simulink model "ac_monitor_A_test"  (R2024b)
settings: Solver=VariableStepAuto  StartTime=0.0  StopTime=80  RelTol=1e-3
PreLoadFcn:
  | load_system('../simulink_reference_models/test_sequence_lib');
InitFcn:
  | close all
  | clear all
  | 
  | T_CNTL = 1/5e3;
  | 
  | VLL_NOM = 35e3;
  | F_NOM = 60;
libraries: test_sequence_lib x4
settings Model: SimulationMode=rapid-accelerator  Creator=HussamAlatrash  LastModifiedBy=ritvik_heron

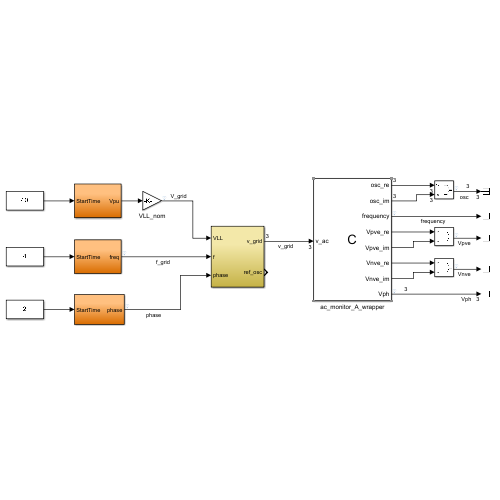
[thumbnail: Simulink's stored preview of the top-level diagram]
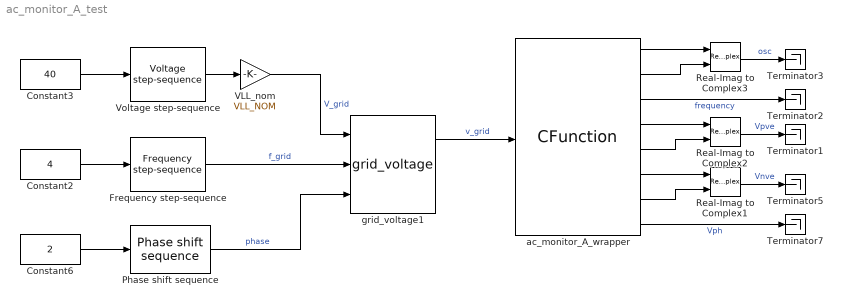
== system ac_monitor_A_test ==
  Constant2 : Constant  Value=4
  Constant3 : Constant  Value=40
  Constant6 : Constant  Value=2
  Frequency step-sequence : test_sequence_lib/Frequency step-sequence  SystemSampleTime=-1  VariantActivationTime=update diagram  AllowFlexibleInterface=on  Latency=0  AutoFrameSizeCalculation=off
  Phase shift sequence : test_sequence_lib/Phase shift sequence  SystemSampleTime=-1  VariantActivationTime=update diagram  AllowFlexibleInterface=on  Latency=0  AutoFrameSizeCalculation=off
  Real-Imag to Complex1 : RealImagToComplex
  Real-Imag to Complex2 : RealImagToComplex
  Real-Imag to Complex3 : RealImagToComplex
  Terminator{1..3,5,7} (5 alike) : Terminator
  VLL_nom : Gain  Gain=VLL_NOM
  Voltage step-sequence : test_sequence_lib/Voltage step-sequence  SystemSampleTime=-1  VariantActivationTime=update diagram  AllowFlexibleInterface=on  Latency=0  AutoFrameSizeCalculation=off
  ac_monitor_A_wrapper : CFunction  OutputCode=|  StartCode=|  CodegenOutputCode=|  CodegenStartCode=|  SampleTime=200e-6  SimCustomHeaderFile=../c_language_library/companion_algorithms/ac_monitor_A/acMonitor_A_autogen.h  SimCustomSourceFile=../c_language_library/companion_algorithms/ac_monitor_A/ac_monitor_A.c ../c_language_library/helper_lib/cmplx.c  CustomHeaderFile=../c_language_library/companion_algorithms/ac_monitor_A/acMonitor_A_autogen.h  CustomSourceFile=../c_language_library/companion_algorithms/ac_monitor_A/ac_monitor_A.c ../c_language_library/helper_lib/cmplx.c
      OutputCode=|
      | acMonitor_IN.v_ac[0] = v_ac[0];
      | acMonitor_IN.v_ac[1] = v_ac[1];
      | acMonitor_IN.v_ac[2] = v_ac[2];
      | 
      | 
      | acMonitor_5kHz(200e-6f);
      | 
      | osc_re[0] = acMonitor_OUT.pll_osc[0].real;
      | osc_im[0] = acMonitor_OUT.pll_osc[0].imag;
      | osc_re[1] = acMonitor_OUT.pll_osc[1].real;
      | osc_im[1] = acMonitor_OUT.pll_osc[1].imag;
      | osc_re[2] = acMonitor_OUT.pll_osc[2].real;
      | osc_im[2] = acMonitor_OUT.pll_osc[2].imag;
      | 
      | frequency = acMonitor_OUT.frequency;
      | Vpve_re = acMonitor_OUT.Vpve.real;
      | Vpve_im = acMonitor_OUT.Vpve.imag;
      | Vnve_re = acMonitor_OUT.Vnve.real;
      | Vnve_im = acMonitor_OUT.Vnve.imag;
      | 
      | Vph[0] = acMonitor_OUT.Vph[0];
      | Vph[1] = acMonitor_OUT.Vph[1];
      | Vph[2] = acMonitor_OUT.Vph[2];
      StartCode=|
      | set_acMonitor_GENERAL_CFG_VllRated(35e3);
      | acMonitor_update_derived_config();
      CodegenOutputCode=|
      | acMonitor_IN.v_ac[0] = v_ac[0];
      | acMonitor_IN.v_ac[1] = v_ac[1];
      | acMonitor_IN.v_ac[2] = v_ac[2];
      | 
      | 
      | acMonitor_5kHz(200e-6f);
      | 
      | osc_re[0] = acMonitor_OUT.pll_osc[0].real;
      | osc_im[0] = acMonitor_OUT.pll_osc[0].imag;
      | osc_re[1] = acMonitor_OUT.pll_osc[1].real;
      | osc_im[1] = acMonitor_OUT.pll_osc[1].imag;
      | osc_re[2] = acMonitor_OUT.pll_osc[2].real;
      | osc_im[2] = acMonitor_OUT.pll_osc[2].imag;
      | 
      | frequency = acMonitor_OUT.frequency;
      | Vpve_re = acMonitor_OUT.Vpve.real;
      | Vpve_im = acMonitor_OUT.Vpve.imag;
      | Vnve_re = acMonitor_OUT.Vnve.real;
      | Vnve_im = acMonitor_OUT.Vnve.imag;
      | 
      | Vph[0] = acMonitor_OUT.Vph[0];
      | Vph[1] = acMonitor_OUT.Vph[1];
      | Vph[2] = acMonitor_OUT.Vph[2];
      CodegenStartCode=|
      | set_acMonitor_GENERAL_CFG_VllRated(35e3);
      | acMonitor_update_derived_config();
  grid_voltage1 : test_sequence_lib/grid_voltage  SystemSampleTime=-1  VariantActivationTime=update diagram  AllowFlexibleInterface=on  Latency=0  AutoFrameSizeCalculation=off
  wires:
  VLL_nom/1 -> grid_voltage1/1  "V_grid"
  Voltage step-sequence/1 -> VLL_nom/1
  Constant3/1 -> Voltage step-sequence/1
  grid_voltage1/1 -> ac_monitor_A_wrapper/1  "v_grid"
  ac_monitor_A_wrapper/1 -> Real-Imag to Complex3/1
  ac_monitor_A_wrapper/2 -> Real-Imag to Complex3/2
  ac_monitor_A_wrapper/3 -> Terminator2/1  "frequency"
  ac_monitor_A_wrapper/4 -> Real-Imag to Complex2/1
  ac_monitor_A_wrapper/5 -> Real-Imag to Complex2/2
  ac_monitor_A_wrapper/6 -> Real-Imag to Complex1/1
  Constant6/1 -> Phase shift sequence/1
  Frequency step-sequence/1 -> grid_voltage1/2  "f_grid"
  Phase shift sequence/1 -> grid_voltage1/3  "phase"
  Constant2/1 -> Frequency step-sequence/1
  ac_monitor_A_wrapper/8 -> Terminator7/1  "Vph"
  ac_monitor_A_wrapper/7 -> Real-Imag to Complex1/2
  Real-Imag to Complex1/1 -> Terminator5/1  "Vnve"
  Real-Imag to Complex2/1 -> Terminator1/1  "Vpve"
  Real-Imag to Complex3/1 -> Terminator3/1  "osc"
